simulink model "q1_e"  (R2025a)
settings: Solver=VariableStepAuto  StartTime=0.0  StopTime=200  RelTol=1e-3
settings Model: Creator=dtemu  LastModifiedBy=dtemu

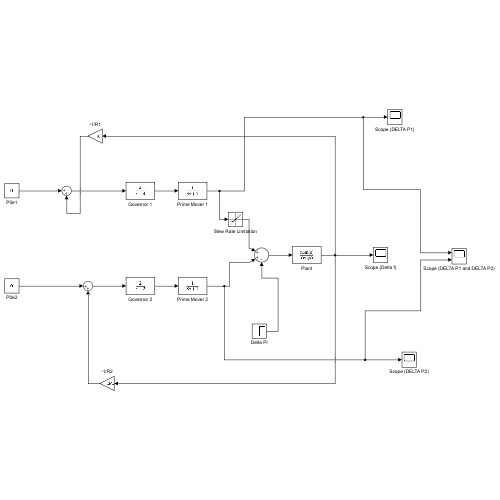
[thumbnail: Simulink's stored preview of the top-level diagram]
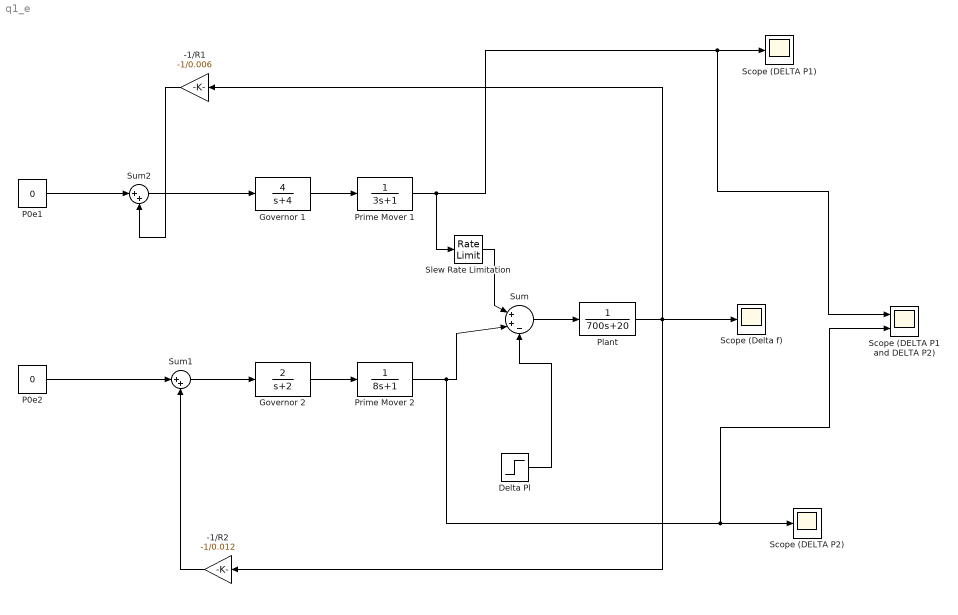
== system q1_e ==
  -1/R1 : Gain  Gain=-1/0.006
  -1/R2 : Gain  Gain=-1/0.012
  Delta Pl : Step  Time=0  After=100  SampleTime=0
  Governor 1 : TransferFcn  Numerator=[4]  Denominator=[1 4]
  Governor 2 : TransferFcn  Numerator=[2]  Denominator=[1 2]
  P0e1 : Constant  Value=0
  P0e2 : Constant  Value=0
  Plant : TransferFcn  Denominator=[700 20]
  Prime Mover 1 : TransferFcn  Denominator=[3 1]
  Prime Mover 2 : TransferFcn  Denominator=[8 1]
  Scope (DELTA P1 and DELTA P2) : Scope  NumInputPorts=2
      settings: ActiveDisplayYMinimum=-5.194362157685589  ActiveDisplayYMaximum=184.30850542084431  DataLoggingVariableName=ScopeData3
  Scope (DELTA P1) : Scope
      settings: ActiveDisplayYMinimum=-36.526749357518838  ActiveDisplayYMaximum=216.61980331125767  DataLoggingVariableName=ScopeData2
  Scope (DELTA P2) : Scope
      settings: ActiveDisplayYMinimum=-6.5608903812980657  ActiveDisplayYMaximum=83.6738834973829
  Scope (Delta f) : Scope
      settings: ActiveDisplayYMinimum=-1.2466318484232528  ActiveDisplayYMaximum=0.13851464982480585
  Slew Rate Limitation : RateLimiter  SampleTimeMode=inherited
  Sum : Sum  Inputs=|++-
  Sum1 : Sum  Inputs=|++
  Sum2 : Sum  Inputs=|++
  wires:
  Prime Mover 1/1 -> Slew Rate Limitation/1, Scope (DELTA P1 and DELTA P2)/1, Scope (DELTA P1)/1
  -1/R1/1 -> Sum2/2
  Governor 2/1 -> Prime Mover 2/1
  Governor 1/1 -> Prime Mover 1/1
  P0e1/1 -> Sum2/1
  Sum/1 -> Plant/1
  Plant/1 -> -1/R1/1, Scope (Delta f)/1, -1/R2/1
  Delta Pl/1 -> Sum/3
  Prime Mover 2/1 -> Scope (DELTA P1 and DELTA P2)/2, Scope (DELTA P2)/1, Sum/2
  -1/R2/1 -> Sum1/2
  P0e2/1 -> Sum1/1
  Sum1/1 -> Governor 2/1
  Sum2/1 -> Governor 1/1
  Slew Rate Limitation/1 -> Sum/1
